simulink model "model"  (R2021a)
settings: Solver=VariableStepAuto  StartTime=0.0  StopTime=10  RelTol=1e-3
values from neighbouring files (symbols this model uses):
  aFront = 2.2    [params.m]
  Bx = 0    [LaneFollowingVehicleModel.m]    (also in jacFunc.m; mainn.m; modelKating.m; modelOutputKating.m)
  By = 0    [LaneFollowingVehicleModel.m]    (also in jacFunc.m; mainn.m; modelKating.m; modelOutputKating.m)
  cAlphaFront = 0.09    [params.m]
  cAlphaR = 0.09    [params.m]
  cDrag = 0.3    [params.m]
  cZigmaFront = 55    [params.m]
  fr = 0.02    [LaneFollowingVehicleModel.m]    (also in jacFunc.m; mainn.m; modelKating.m; modelOutputKating.m)
  g = 9.81    [LaneFollowingVehicleModel.m]    (also in jacFunc.m; mainn.m; modelKating.m; modelOutputKating.m)
  Iz = 1536.70    (= 1536.7)    [LaneFollowingVehicleModel.m]    (also in jacFunc.m; mainn.m; modelKating.m; modelOutputKating.m)
  lf = 1.22    [LaneFollowingVehicleModel.m]    (also in jacFunc.m; mainn.m; modelKating.m; modelOutputKating.m)
  lr = 1.36    [LaneFollowingVehicleModel.m]    (also in jacFunc.m; mainn.m; modelKating.m; modelOutputKating.m)
  m = 1500 + 2*80 + 300    (= 1960)    [LaneFollowingVehicleModel.m]    (also in jacFunc.m; mainn.m; modelKating.m; modelOutputKating.m)
  reff = sin(B)/B * rnom    [LaneFollowingVehicleModel.m]    (also in jacFunc.m; mainn.m; modelKating.m; modelOutputKating.m)
  rhoAir = 1.225    [params.m]
libraries: mpclib x1
settings Model: Creator=septi  LastModifiedBy=septi

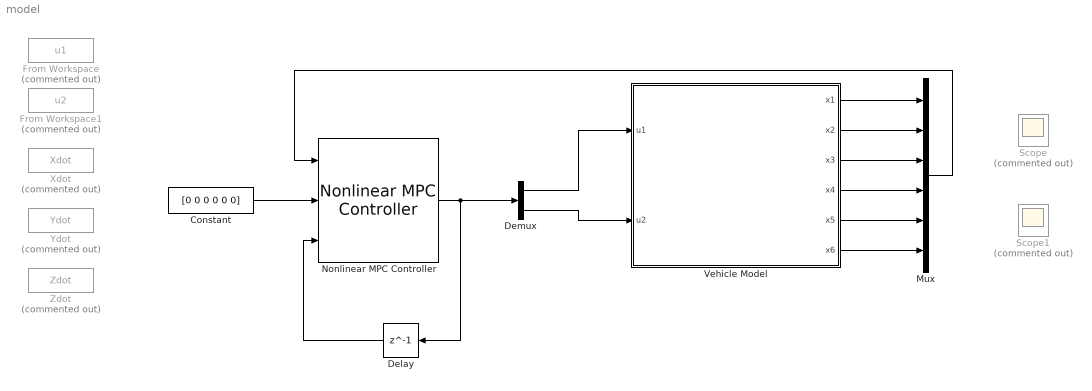
== system model ==
  Constant : Constant  Value=[0 0 0 0 0 0]  VectorParams1D=off
  Delay : Delay  DelayLength=1  InitialCondition=[0.2 0.3]
  Demux : Demux  Outputs=2
  From Workspace : FromWorkspace  Commented=on  VariableName=u1
  From Workspace1 : FromWorkspace  Commented=on  VariableName=u2
  Mux : Mux  Inputs=6
  Nonlinear MPC Controller : mpclib/Nonlinear MPC Controller  SCDEnableBlockLinearizationSpecification=on  nlmpcobj=nlobj  UseObjectTs=on  UseMEX=off  md_enabled=off  mvtarget_enabled=off  param_enabled=off  cost_enabled=off  mvseq_enabled=off  stateseq_enabled=off  ovseq_enabled=off  slack_enabled=off  status_enabled=off  ov_min=off  ov_max=off  mv_min=off  mv_max=off  mvrate_min=off  mvrate_max=off  state_min=off  state_max=off  ov_weight=off  mv_weight=off  mvrate_weight=off  ecr_weight=off  nlp_initialize=off
  Scope : Scope  Commented=on
  Scope1 : Scope  Commented=on
  Vehicle Model : Subsystem
  Xdot : FromWorkspace  Commented=on  VariableName=Xdot
  Ydot : FromWorkspace  Commented=on  VariableName=Ydot
  Zdot : FromWorkspace  Commented=on  VariableName=Zdot
  wires:
  Nonlinear MPC Controller/1 -> Demux/1, Delay/1
  Delay/1 -> Nonlinear MPC Controller/3
  Demux/1 -> Vehicle Model/1(u1)
  Demux/2 -> Vehicle Model/2(u2)
  Vehicle Model/1(x1) -> Mux/1
  Vehicle Model/2(x2) -> Mux/2
  Vehicle Model/3(x3) -> Mux/3
  Vehicle Model/4(x4) -> Mux/4
  Vehicle Model/5(x5) -> Mux/5
  Vehicle Model/6(x6) -> Mux/6
  Mux/1 -> Nonlinear MPC Controller/1
  Constant/1 -> Nonlinear MPC Controller/2

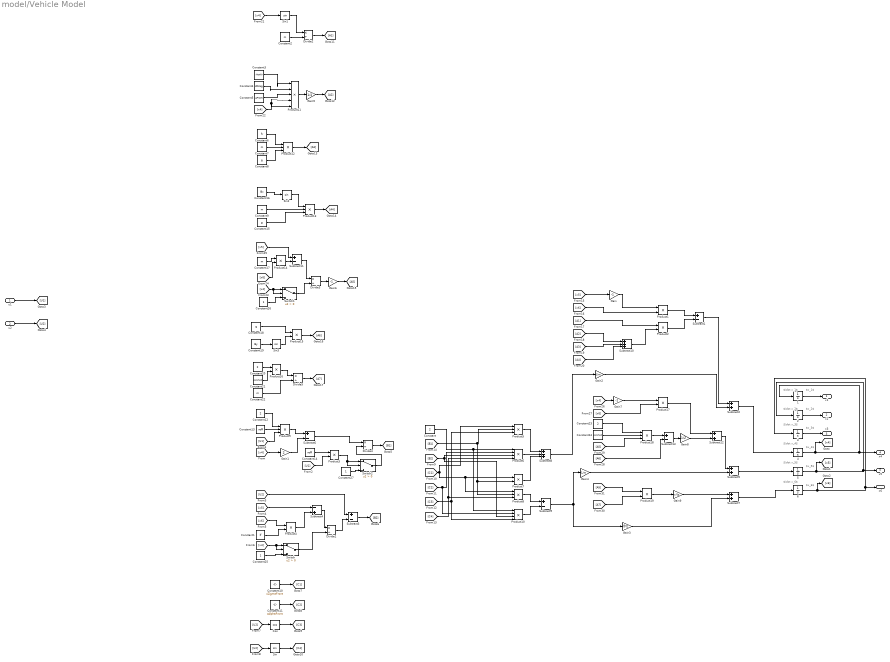
== system model/Vehicle Model ==
  note: $x_1$
  note: $x_2$
  note: $x_3$
  note: $x_4$
  note: $x_5$
  note: $x_6$
  note: $\dot x_1$
  note: $\dot x_2$
  note: $\dot x_6$
  note: $\dot x_4$
  note: $\dot x_3$
  note: $\dot x_5$
  u1 : Inport
  u2 : Inport  Port=2
  {1..6} (6 alike) : Integrator
  Constant{,12,20,23} (4 alike) : Constant  Value=2
  Constant1 : Constant  Value=lf
  Constant10 : Constant  Value=cZigmaFront
  Constant11 : Constant  Value=cAlphaFront
  Constant13 : Constant  Value=reff
  Constant14 : Constant  Value=reff
  Constant15 : Constant  Value=g
  Constant16 : Constant  Value=Bx
  Constant{2,7,9,17,22} (5 alike) : Constant  Value=m
  Constant18 : Constant  Value=g
  Constant19 : Constant  Value=By
  Constant21 : Constant  Value=cAlphaR
  Constant24 : Constant  Value=cAlphaR
  Constant25 : Constant
  Constant26 : Constant
  Constant27 : Constant
  Constant3 : Constant  Value=rhoAir
  Constant4 : Constant  Value=cDrag
  Constant5 : Constant  Value=aFront
  Constant6 : Constant  Value=fr
  Constant8 : Constant  Value=g
  Cos : Trigonometry  Operator=cos
  Divide{1..5} (5 alike) : Product  Inputs=*/
  Gain : Gain  Gain=-1
  Gain1 : Gain  Gain=2
  Gain2 : Gain  Gain=1/m
  Gain3 : Gain  Gain=lf/Iz
  Gain4 : Gain  Gain=1/m
  Gain5 : Gain  Gain=1/2
  Gain6 : Gain  Gain=-1
  Gain7 : Gain  Gain=-1
  Gain8 : Gain  Gain=1/2
  Gain9 : Gain  Gain=lr/Iz
  Product{1..4,7,14..17,19} (10 alike) : Product
  Product10 : Product  Inputs=4
  Product11 : Product  Inputs=5
  Product{5,8..9,12..13,18} (6 alike) : Product  Inputs=3
  Product6 : Product  Inputs=4
  Sin{,1..3} (4 alike) : Trigonometry
  Subtract{1,3,6,9,11,13} (6 alike) : Sum  Inputs=+-
  Subtract10 : Sum  Inputs=+++
  Subtract{2,5,7,12} (4 alike) : Sum
  Subtract4 : Sum  Inputs=-+
  Subtract8 : Sum  Inputs=+-+
  Switch : Switch  Criteria=u2 > Threshold
  Switch1 : Switch  Criteria=u2 > Threshold
  Switch2 : Switch  Criteria=u2 > Threshold
  x1 : Outport
  x2 : Outport  Port=2
  x3 : Outport  Port=3
  x4 : Outport  Port=4
  x5 : Outport  Port=5
  x6 : Outport  Port=6
  wires:
  Product4/1 -> Subtract4/2
  Constant8/1 -> Product12/3
  Product18/1 -> Subtract13/1
  Subtract12/1 -> Subtract5/1
  [x4] -> Gain1/1
  [A2] -> Subtract10/1
  Subtract9/1 -> Gain3/1, Gain4/1
  Switch/1 -> Divide1/2
  Divide4/1 -> [B1]
  [B1] -> Product7/2, Product8/2, Product5/2
  Product7/1 -> Subtract8/3
  [A5] -> Product19/1
  Constant25/1 -> Switch/3
  Product6/1 -> Subtract8/2
  Constant16/1 -> Sin2/1
  Gain9/1 -> Subtract7/1
  [x6] -> Product17/2
  Subtract6/1 -> Divide4/1
  6/1 -> [x6], x6/1, 3/1
  Switch2/1 -> Divide4/2
  Subtract13/1 -> Gain8/1
  u2/1 -> [U2]
  [x4] -> Switch/2, Switch/1
  Product12/1 -> [A3]
  Constant24/1 -> Product18/2
  Constant18/1 -> Product15/1
  Product16/1 -> Divide5/1
  Subtract5/1 -> 5/1
  [x5] -> Subtract4/1
  [A5] -> Product18/3
  Constant23/1 -> Product18/1
  Gain2/1 -> Subtract2/2
  Constant/1 -> Product10/1, Product6/1
  Product10/1 -> Subtract9/2
  Constant14/1 -> Product3/1
  Switch1/1 -> Divide3/2
  [U2] -> Cos/1
  Constant5/1 -> Product11/3
  Constant6/1 -> Product12/1
  [C1] -> Product8/1, Product7/1, Product5/1
  Product15/1 -> [A6]
  5/1 -> [x5], x5/1, 2/1
  Divide2/1 -> [A1]
  Subtract11/1 -> Divide3/1
  Constant26/1 -> Switch1/3
  Product11/1 -> Gain5/1
  [x4] -> Switch1/2, Switch1/1
  4/1 -> [x4], x4/1, 1/1
  Product3/1 -> Switch2/2, Switch2/1
  [U1] -> Product3/2
  Gain1/1 -> Subtract6/2
  [x4] -> Product11/5, Product11/4
  Constant27/1 -> Switch2/3
  Gain8/1 -> Subtract12/2
  Constant22/1 -> Divide5/2
  Product8/1 -> Subtract9/1
  [A7] -> Product19/2
  Constant13/1 -> Product9/2
  Constant10/1 -> [C1]
  Gain4/1 -> Subtract5/2
  [x6] -> Product4/1
  Product19/1 -> Gain9/1
  [x5] -> Subtract11/1
  [x5] -> Gain/1
  Gain6/1 -> [A5]
  Constant1/1 -> Product4/2
  Gain3/1 -> Subtract7/2
  Subtract7/1 -> 6/1
  Constant21/1 -> Product16/2
  Divide1/1 -> Subtract3/2
  [C3] -> Product10/4, Product5/3
  Subtract3/1 -> [B2]
  [C2] -> Product10/2, Product6/2
  Constant11/1 -> [C2]
  Sin/1 -> [C4]
  Divide3/1 -> Gain6/1
  Cos/1 -> [C3]
  [U2] -> Subtract3/1
  Subtract2/1 -> 4/1
  [C4] -> Product8/3, Product6/4
  [A3] -> Subtract10/2
  Product1/1 -> Subtract1/1
  [U1] -> Product9/3
  [A4] -> Subtract10/3
  Subtract1/1 -> Subtract2/1
  Sin1/1 -> Divide2/1
  [x6] -> Product1/2
  Gain/1 -> Product1/1
  Constant9/1 -> Product13/2
  [A1] -> Product2/1
  Product9/1 -> Subtract6/1
  Gain5/1 -> [A2]
  [U2] -> Sin/1
  Subtract10/1 -> Product2/2
  Constant3/1 -> Product11/1
  Constant7/1 -> Product12/2
  Sin2/1 -> Product13/1
  Product5/1 -> Subtract8/1
  Constant12/1 -> Product9/1
  Constant2/1 -> Divide2/2
  [x6] -> Product14/2
  Product13/1 -> [A4]
  [B2] -> Product10/3, Product6/3
  Constant17/1 -> Product14/1
  [x4] -> Sin1/1
  Subtract8/1 -> Gain2/1
  Sin3/1 -> Product15/2
  Constant19/1 -> Sin3/1
  Product14/1 -> Subtract11/2
  Subtract4/1 -> Divide1/1
  [x4] -> Gain7/1
  Gain7/1 -> Product17/1
  Constant4/1 -> Product11/2
  Constant15/1 -> Product13/3
  Product17/1 -> Subtract12/1
  Constant20/1 -> Product16/1
  Divide5/1 -> [A7]
  Product2/1 -> Subtract1/2
  [A6] -> Subtract13/2
  u1/1 -> [U1]
  1/1 -> x1/1
  2/1 -> x2/1
  3/1 -> x3/1
